simulink model "Stepper_Model_HIL"  (R2017a)
settings: Solver=FixedStepAuto  StartTime=0.0  StopTime=20  FixedStep=T  RelTol=1e-3
undefined symbols (not defined in the file): Ad, Bd, Cd, Dd, Ptheta0, T
libraries: instrumentlib x8, simulink x2
settings Model: Creator=Patrick  LastModifiedBy=Patrick

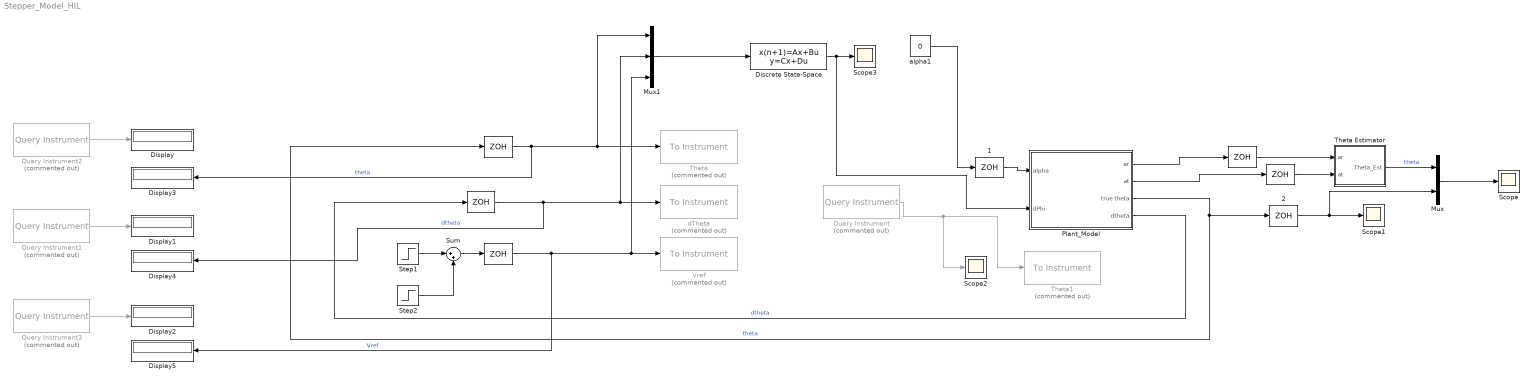
== system Stepper_Model_HIL ==
  " " : ZeroOrderHold  SampleTime=T
  "   " : ZeroOrderHold  SampleTime=T
  "    " : ZeroOrderHold  SampleTime=T
  "      " : ZeroOrderHold  SampleTime=T
  "        " : ZeroOrderHold  SampleTime=T
  "      1" : ZeroOrderHold  SampleTime=T
  "      2" : ZeroOrderHold  SampleTime=T
  Discrete State-Space : DiscreteStateSpace  A=Ad  B=Bd  C=Cd  D=Dd  SampleTime=T
  Display{,1..5} (6 alike) : Display
  Mux : Mux  Inputs=2
  Mux1 : Mux  Inputs=3
  Plant_Model : Subsystem
  Query Instrument : instrumentlib/Query Instrument  Priority=7  Commented=on  sampleTime=T  isWorkspaceObject=off  timeout=10  inputBufferSize=512  protocol=Serial  serialPort=COM4  baudRate=115200  gpibVendor=Agilent Technologies  boardIndex=0  primaryAddress=1  secondaryAddress=0  visaVendor=Agilent  visaSerialPort=0  chassisIndex=0  logicalAddress=0  tcpRemoteHost='127.0.0.1'  tcpRemotePort=4500  udpRemoteHost='127.0.0.1'  udpRemotePort=9090  visaTCPBoardIndex=0  visaTCPRemoteHost='127.0.0.1'  usbBoardIndex=0  usbManufID=0  usbModelCode=0  usbSerialNumber=0  initAction=None  initCommand='DATA:SOURCE CH1'  initFunction=get  queryCommand='ctrl'  responseFormat=ASCII  asciiFormatting='%g\n'  precision=8-bit integer  byteOrder=Little endian  valuesToRead=1  removeBytes=off  afterOutputAction=Repeat query for new data  enableFrames=off  frameSize=1
      settings: SourceProductName=Instrument Control Toolbox  SourceProductBaseCode=IC
  Query Instrument1 : instrumentlib/Query Instrument  Priority=5  Commented=on  sampleTime=T  isWorkspaceObject=off  timeout=10  inputBufferSize=512  protocol=Serial  serialPort=COM4  baudRate=115200  gpibVendor=Agilent Technologies  boardIndex=0  primaryAddress=1  secondaryAddress=0  visaVendor=Agilent  visaSerialPort=0  chassisIndex=0  logicalAddress=0  tcpRemoteHost='127.0.0.1'  tcpRemotePort=4500  udpRemoteHost='127.0.0.1'  udpRemotePort=9090  visaTCPBoardIndex=0  visaTCPRemoteHost='127.0.0.1'  usbBoardIndex=0  usbManufID=0  usbModelCode=0  usbSerialNumber=0  initAction=None  initCommand='DATA:SOURCE CH1'  initFunction=get  queryCommand='dtheta'  responseFormat=ASCII  asciiFormatting='%g\n'  precision=8-bit integer  byteOrder=Little endian  valuesToRead=1  removeBytes=off  afterOutputAction=Repeat query for new data  enableFrames=off  frameSize=1
      settings: SourceProductName=Instrument Control Toolbox  SourceProductBaseCode=IC
  Query Instrument2 : instrumentlib/Query Instrument  Priority=4  Commented=on  sampleTime=T  isWorkspaceObject=off  timeout=10  inputBufferSize=512  protocol=Serial  serialPort=COM4  baudRate=115200  gpibVendor=Agilent Technologies  boardIndex=0  primaryAddress=1  secondaryAddress=0  visaVendor=Agilent  visaSerialPort=0  chassisIndex=0  logicalAddress=0  tcpRemoteHost='127.0.0.1'  tcpRemotePort=4500  udpRemoteHost='127.0.0.1'  udpRemotePort=9090  visaTCPBoardIndex=0  visaTCPRemoteHost='127.0.0.1'  usbBoardIndex=0  usbManufID=0  usbModelCode=0  usbSerialNumber=0  initAction=None  initCommand='DATA:SOURCE CH1'  initFunction=get  queryCommand='theta'  responseFormat=ASCII  asciiFormatting='%g\n'  precision=8-bit integer  byteOrder=Little endian  valuesToRead=1  removeBytes=off  afterOutputAction=Repeat query for new data  enableFrames=off  frameSize=1
      settings: SourceProductName=Instrument Control Toolbox  SourceProductBaseCode=IC
  Query Instrument3 : instrumentlib/Query Instrument  Priority=6  Commented=on  sampleTime=T  isWorkspaceObject=off  timeout=10  inputBufferSize=512  protocol=Serial  serialPort=COM4  baudRate=115200  gpibVendor=Agilent Technologies  boardIndex=0  primaryAddress=1  secondaryAddress=0  visaVendor=Agilent  visaSerialPort=0  chassisIndex=0  logicalAddress=0  tcpRemoteHost='127.0.0.1'  tcpRemotePort=4500  udpRemoteHost='127.0.0.1'  udpRemotePort=9090  visaTCPBoardIndex=0  visaTCPRemoteHost='127.0.0.1'  usbBoardIndex=0  usbManufID=0  usbModelCode=0  usbSerialNumber=0  initAction=None  initCommand='DATA:SOURCE CH1'  initFunction=get  queryCommand='vref'  responseFormat=ASCII  asciiFormatting='%g\n'  precision=8-bit integer  byteOrder=Little endian  valuesToRead=1  removeBytes=off  afterOutputAction=Repeat query for new data  enableFrames=off  frameSize=1
      settings: SourceProductName=Instrument Control Toolbox  SourceProductBaseCode=IC
  Scope{,1..3} (4 alike) : Scope
  Step1 : Step  Time=0  After=-.5  SampleTime=0
  Step2 : Step  Time=5  After=.5  SampleTime=0
  Sum : Sum  Inputs=|++
  Theta : instrumentlib/To Instrument  Priority=1  Commented=on  sampleTime=T  isWorkspaceObject=off  timeout=10  inputBufferSize=8192  protocol=Serial  serialPort=COM4  baudRate=115200  gpibVendor=Agilent Technologies  boardIndex=0  primaryAddress=1  secondaryAddress=0  visaVendor=Agilent  visaSerialPort=0  chassisIndex=0  logicalAddress=0  tcpRemoteHost='127.0.0.1'  tcpRemotePort=4500  udpRemoteHost='127.0.0.1'  udpRemotePort=9090  visaTCPBoardIndex=0  visaTCPRemoteHost='127.0.0.1'  usbBoardIndex=0  usbManufID=0  usbModelCode=0  usbSerialNumber=0  initAction=None  initCommand='DATA:SOURCE CH1'  initFunction=get  command=''  sendFormat=ASCII  asciiFormatting='set theta %g\n'  precision=8-bit integer  byteOrder=Little endian
      settings: SourceProductName=Instrument Control Toolbox  SourceProductBaseCode=IC
  Theta Estimator : Subsystem
  Theta1 : instrumentlib/To Instrument  Priority=8  Commented=on  sampleTime=T  isWorkspaceObject=off  timeout=10  inputBufferSize=8192  protocol=Serial  serialPort=COM4  baudRate=115200  gpibVendor=Agilent Technologies  boardIndex=0  primaryAddress=1  secondaryAddress=0  visaVendor=Agilent  visaSerialPort=0  chassisIndex=0  logicalAddress=0  tcpRemoteHost='127.0.0.1'  tcpRemotePort=4500  udpRemoteHost='127.0.0.1'  udpRemotePort=9090  visaTCPBoardIndex=0  visaTCPRemoteHost='127.0.0.1'  usbBoardIndex=0  usbManufID=0  usbModelCode=0  usbSerialNumber=0  initAction=None  initCommand='DATA:SOURCE CH1'  initFunction=get  command=''  sendFormat=ASCII  asciiFormatting='motor speed %g\n'  precision=8-bit integer  byteOrder=Little endian
      settings: SourceProductName=Instrument Control Toolbox  SourceProductBaseCode=IC
  Vref : instrumentlib/To Instrument  Priority=3  Commented=on  sampleTime=T  isWorkspaceObject=off  timeout=10  inputBufferSize=8192  protocol=Serial  serialPort=COM4  baudRate=115200  gpibVendor=Agilent Technologies  boardIndex=0  primaryAddress=1  secondaryAddress=0  visaVendor=Agilent  visaSerialPort=0  chassisIndex=0  logicalAddress=0  tcpRemoteHost='127.0.0.1'  tcpRemotePort=4500  udpRemoteHost='127.0.0.1'  udpRemotePort=9090  visaTCPBoardIndex=0  visaTCPRemoteHost='127.0.0.1'  usbBoardIndex=0  usbManufID=0  usbModelCode=0  usbSerialNumber=0  initAction=None  initCommand='DATA:SOURCE CH1'  initFunction=get  command=''  sendFormat=ASCII  asciiFormatting='set vref %g\n'  precision=8-bit integer  byteOrder=Little endian
      settings: SourceProductName=Instrument Control Toolbox  SourceProductBaseCode=IC
  alpha1 : Constant  Value=0
  dTheta : instrumentlib/To Instrument  Priority=2  Commented=on  sampleTime=T  isWorkspaceObject=off  timeout=10  inputBufferSize=8192  protocol=Serial  serialPort=COM4  baudRate=115200  gpibVendor=Agilent Technologies  boardIndex=0  primaryAddress=1  secondaryAddress=0  visaVendor=Agilent  visaSerialPort=0  chassisIndex=0  logicalAddress=0  tcpRemoteHost='127.0.0.1'  tcpRemotePort=4500  udpRemoteHost='127.0.0.1'  udpRemotePort=9090  visaTCPBoardIndex=0  visaTCPRemoteHost='127.0.0.1'  usbBoardIndex=0  usbManufID=0  usbModelCode=0  usbSerialNumber=0  initAction=None  initCommand='DATA:SOURCE CH1'  initFunction=get  command=''  sendFormat=ASCII  asciiFormatting='set dtheta %g\n'  precision=8-bit integer  byteOrder=Little endian
      settings: SourceProductName=Instrument Control Toolbox  SourceProductBaseCode=IC
  wires:
  Mux/1 -> Scope/1
  "      "/1 -> Display3/1, Mux1/1, Theta/1  "theta"
  "    "/1 -> Display5/1, Mux1/3, Vref/1  "Vref"
  Plant_Model/1(ar) -> "   "/1
  "   "/1 -> Theta Estimator/1(ar)
  " "/1 -> Theta Estimator/2(at)
  Plant_Model/2(at) -> " "/1
  Theta Estimator/1(Theta_Est) -> Mux/1  "theta"
  Plant_Model/4(dtheta) -> "        "/1  "dtheta"
  Plant_Model/3(true theta) -> "      2"/1, "      "/1  "theta"
  "        "/1 -> Display4/1, Mux1/2, dTheta/1  "dtheta"
  Query Instrument/1 -> Scope2/1, Theta1/1
  "      1"/1 -> Plant_Model/1("alpha ")
  alpha1/1 -> "      1"/1
  "      2"/1 -> Mux/2, Scope1/1
  Query Instrument1/1 -> Display1/1
  Query Instrument2/1 -> Display/1
  Query Instrument3/1 -> Display2/1
  Sum/1 -> "    "/1
  Step1/1 -> Sum/1
  Step2/1 -> Sum/2
  Mux1/1 -> Discrete State-Space/1
  Discrete State-Space/1 -> Plant_Model/2(dPhi), Scope3/1

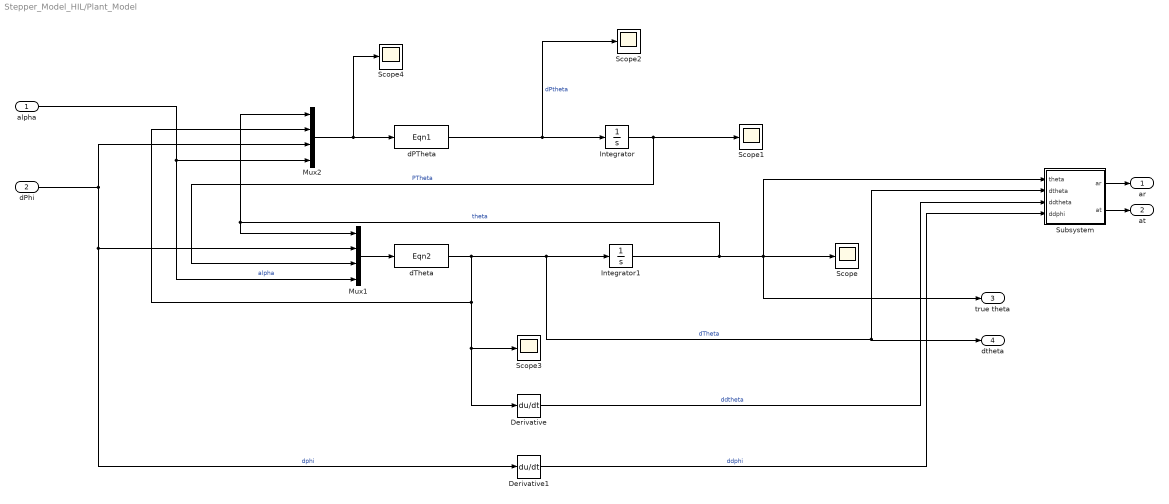
== system Stepper_Model_HIL/Plant_Model ==
  "alpha " : Inport
  dPhi : Inport  Port=2
  Derivative : Derivative
  Derivative1 : Derivative
  Integrator : Integrator  InitialCondition=Ptheta0
  Integrator1 : Integrator  InitialCondition=0.1
  Mux1 : Mux  Inputs=[1 1 1 1]
  Mux2 : Mux  Inputs=[1 1 1 1]
  Scope{,1..4} (5 alike) : Scope
  Subsystem : Subsystem
  dPTheta : MATLABFcn  MATLABFcn=Eqn1  OutputDimensions=[1 1]  Output1D=off
  dTheta : MATLABFcn  MATLABFcn=Eqn2  OutputDimensions=[1 1]  Output1D=off
  ar : Outport  PortDimensions=[1 1]
  at : Outport  Port=2  PortDimensions=[1 1]
  true theta : Outport  Port=3  PortDimensions=[1 1]
  dtheta : Outport  Port=4  PortDimensions=[1 1]
  wires:
  Integrator/1 -> Scope1/1, Mux1/3  "PTheta"
  dPhi/1 -> Mux2/3, Derivative1/1, Mux1/2  "dphi"
  dPTheta/1 -> Integrator/1, Scope2/1  "dPtheta"
  dTheta/1 -> Derivative/1, Scope3/1, Mux2/2, Subsystem/2(dtheta), dtheta/1, Integrator1/1  "dTheta"
  Mux2/1 -> Scope4/1, dPTheta/1
  Mux1/1 -> dTheta/1
  "alpha "/1 -> Mux1/4, Mux2/4  "alpha"
  Derivative/1 -> Subsystem/3(ddtheta)  "ddtheta"
  Derivative1/1 -> Subsystem/4(ddphi)  "ddphi"
  Subsystem/1(ar) -> ar/1
  Subsystem/2(at) -> at/1
  Integrator1/1 -> Mux2/1, Mux1/1, Subsystem/1(theta), true theta/1, Scope/1  "theta"

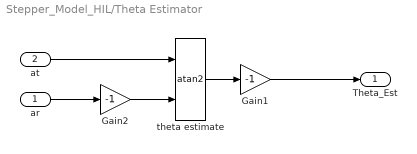
== system Stepper_Model_HIL/Theta Estimator ==
  ar : Inport
  at : Inport  Port=2
  Gain1 : Gain  Gain=-1
  Gain2 : Gain  Gain=-1
  theta estimate : Trigonometry  Operator=atan2  OutputSignalType=real
  Theta_Est : Outport
  wires:
  ar/1 -> Gain2/1
  at/1 -> theta estimate/1
  Gain2/1 -> theta estimate/2
  theta estimate/1 -> Gain1/1
  Gain1/1 -> Theta_Est/1

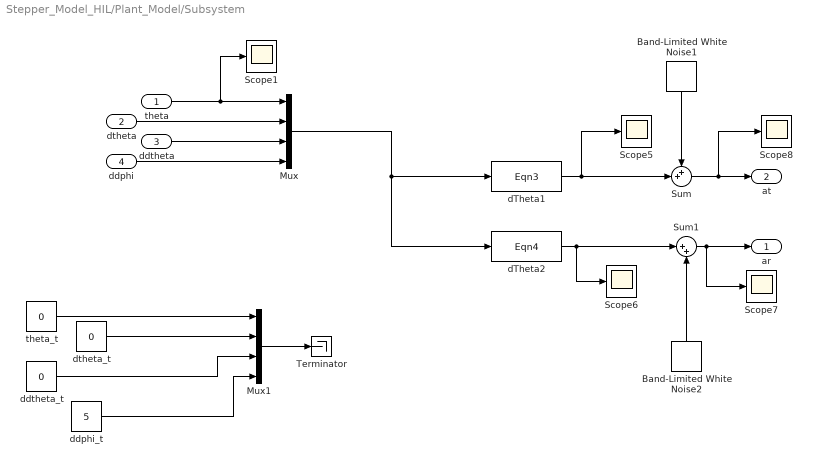
== system Stepper_Model_HIL/Plant_Model/Subsystem ==
  theta : Inport
  dtheta : Inport  Port=2
  ddtheta : Inport  Port=3
  ddphi : Inport  Port=4
  Band-Limited White Noise1 : simulink/Sources/Band-Limited White Noise  Cov=[0.0000001]  Ts=.01  seed=[23341]
  Band-Limited White Noise2 : simulink/Sources/Band-Limited White Noise  Cov=[0.0000001]  Ts=.01  seed=[23341]
  Mux : Mux
  Mux1 : Mux
  Scope{1,5..8} (5 alike) : Scope
  Sum : Sum  Inputs=++|
  Sum1 : Sum  Inputs=|++
  Terminator : Terminator
  dTheta1 : MATLABFcn  MATLABFcn=Eqn3  OutputDimensions=[1 1]  Output1D=off
  dTheta2 : MATLABFcn  MATLABFcn=Eqn4  OutputDimensions=[1 1]  Output1D=off
  ddphi_t : Constant  Value=5
  ddtheta_t : Constant  Value=0
  dtheta_t : Constant  Value=0
  theta_t : Constant  Value=0
  ar : Outport  PortDimensions=[1 1]
  at : Outport  Port=2  PortDimensions=[1 1]
  wires:
  theta/1 -> Scope1/1, Mux/1
  dtheta/1 -> Mux/2
  Sum/1 -> at/1, Scope8/1
  dTheta2/1 -> Sum1/1, Scope6/1
  Sum1/1 -> ar/1, Scope7/1
  dTheta1/1 -> Sum/2, Scope5/1
  ddphi/1 -> Mux/4
  ddtheta/1 -> Mux/3
  Band-Limited White Noise1/1 -> Sum/1
  Band-Limited White Noise2/1 -> Sum1/2
  ddphi_t/1 -> Mux1/4
  theta_t/1 -> Mux1/1
  dtheta_t/1 -> Mux1/2
  ddtheta_t/1 -> Mux1/3
  Mux/1 -> dTheta1/1, dTheta2/1
  Mux1/1 -> Terminator/1
